simulink model "TourismusdynamikSim"  (R2022b)
settings: Solver=VariableStepAuto  StartTime=0.0  StopTime=10.0  RelTol=1e-3
settings Model: Creator=benja  LastModifiedBy=benja

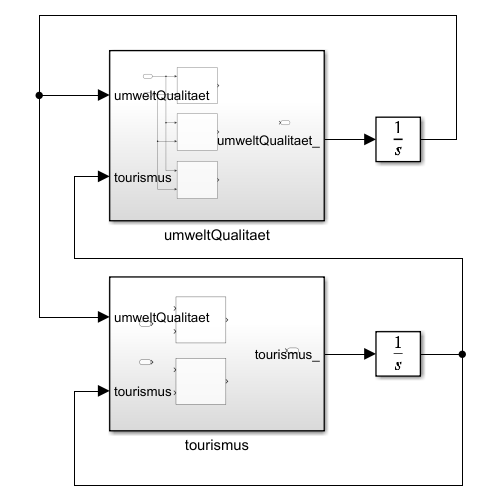
[thumbnail: Simulink's stored preview of the top-level diagram]
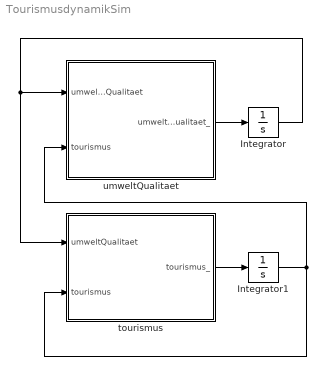
== system TourismusdynamikSim ==
  Integrator : Integrator
  Integrator1 : Integrator
  tourismus : Subsystem
  umweltQualitaet : Subsystem
  wires:
  umweltQualitaet/1(umweltQualitaet_) -> Integrator/1
  tourismus/1(tourismus_) -> Integrator1/1
  Integrator1/1 -> tourismus/2(tourismus), umweltQualitaet/2(tourismus)
  Integrator/1 -> umweltQualitaet/1(umweltQualitaet), tourismus/1(umweltQualitaet)

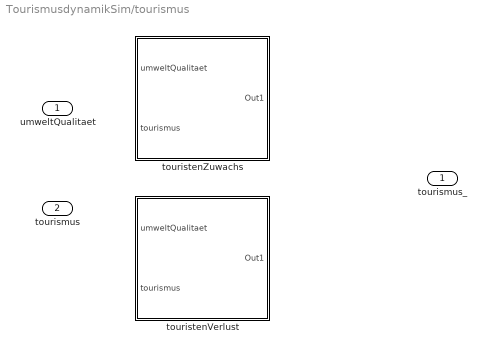
== system TourismusdynamikSim/tourismus ==
  umweltQualitaet : Inport
  tourismus : Inport  Port=2
  touristenVerlust : Subsystem
  touristenZuwachs : Subsystem
  tourismus_ : Outport

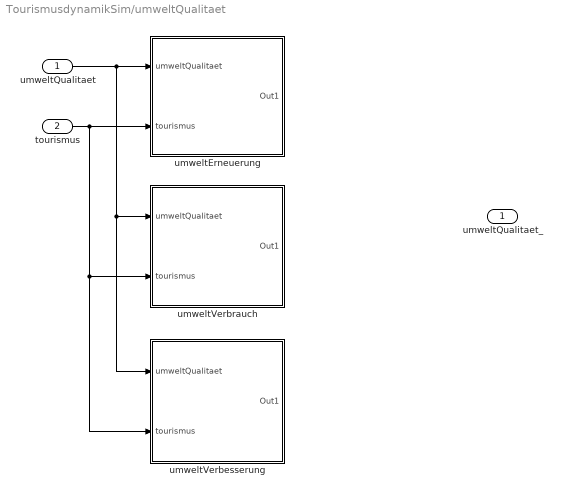
== system TourismusdynamikSim/umweltQualitaet ==
  umweltQualitaet : Inport
  tourismus : Inport  Port=2
  umweltErneuerung : Subsystem
  umweltVerbesserung : Subsystem
  umweltVerbrauch : Subsystem
  umweltQualitaet_ : Outport
  wires:
  umweltQualitaet/1 -> umweltVerbesserung/1(umweltQualitaet), umweltVerbrauch/1(umweltQualitaet), umweltErneuerung/1(umweltQualitaet)
  tourismus/1 -> umweltVerbesserung/2(tourismus), umweltVerbrauch/2(tourismus), umweltErneuerung/2(tourismus)

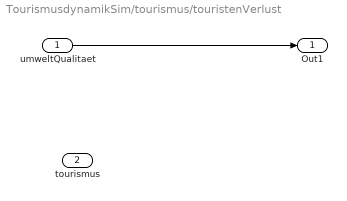
== system TourismusdynamikSim/tourismus/touristenVerlust ==
  umweltQualitaet : Inport
  tourismus : Inport  Port=2
  Out1 : Outport
  wires:
  umweltQualitaet/1 -> Out1/1

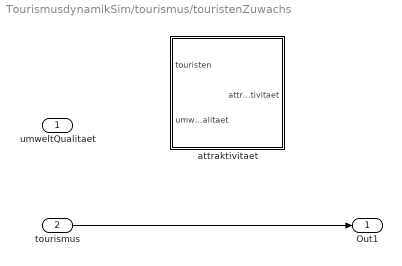
== system TourismusdynamikSim/tourismus/touristenZuwachs ==
  umweltQualitaet : Inport
  tourismus : Inport  Port=2
  attraktivitaet : Subsystem
  Out1 : Outport
  wires:
  tourismus/1 -> Out1/1

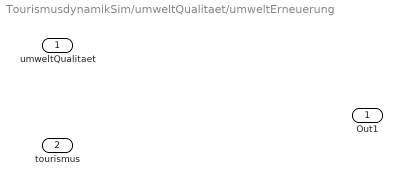
== system TourismusdynamikSim/umweltQualitaet/umweltErneuerung ==
  umweltQualitaet : Inport
  tourismus : Inport  Port=2
  Out1 : Outport

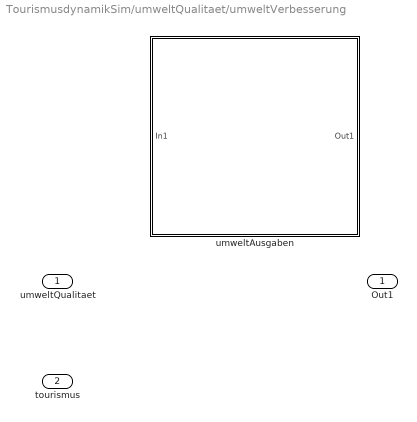
== system TourismusdynamikSim/umweltQualitaet/umweltVerbesserung ==
  umweltQualitaet : Inport
  tourismus : Inport  Port=2
  umweltAusgaben : Subsystem
  Out1 : Outport

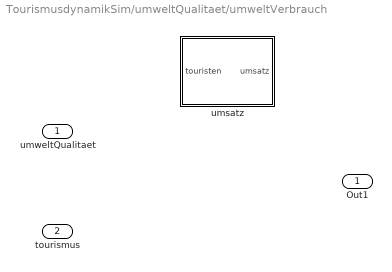
== system TourismusdynamikSim/umweltQualitaet/umweltVerbrauch ==
  umweltQualitaet : Inport
  tourismus : Inport  Port=2
  umsatz : Subsystem
  Out1 : Outport

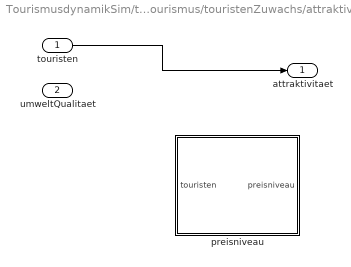
== system TourismusdynamikSim/tourismus/touristenZuwachs/attraktivitaet ==
  touristen : Inport
  umweltQualitaet : Inport  Port=2
  preisniveau : Subsystem
  attraktivitaet : Outport
  wires:
  touristen/1 -> attraktivitaet/1

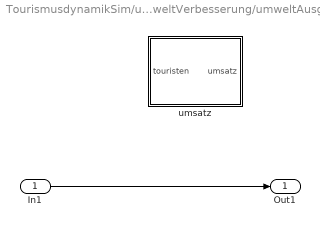
== system TourismusdynamikSim/umweltQualitaet/umweltVerbesserung/umweltAusgaben ==
  In1 : Inport
  umsatz : Subsystem
  Out1 : Outport
  wires:
  In1/1 -> Out1/1

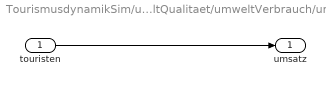
== system TourismusdynamikSim/umweltQualitaet/umweltVerbrauch/umsatz ==
  touristen : Inport
  umsatz : Outport
  wires:
  touristen/1 -> umsatz/1

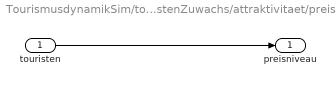
== system TourismusdynamikSim/tourismus/touristenZuwachs/attraktivitaet/preisniveau ==
  touristen : Inport
  preisniveau : Outport
  wires:
  touristen/1 -> preisniveau/1

== system TourismusdynamikSim/umweltQualitaet/umweltVerbesserung/umweltAusgaben/umsatz ==
  touristen : Inport
  umsatz : Outport
  wires:
  touristen/1 -> umsatz/1
